simulink model "FaultCheck"  (R2022b)
settings: Solver=FixedStepAuto  StartTime=0.0  StopTime=10  FixedStep=1  RelTol=1e-3
undefined symbols (not defined in the file): C_Flt_IGBTULowerTempConfirmTh_u16, C_Flt_IGBTULowerTempDiagEn_b, C_Flt_IGBTULowerTempErrCode_u16, C_Flt_IGBTULowerTempPowerCoeff, C_Flt_IGBTULowerTempRecoveryTh_u16, C_Flt_IGBTULowerTempRecTh_s32, C_Flt_IGBTULowerTempTrigTh_s32, C_Flt_IGBTUOverTempConfirmTh_u16, C_Flt_IGBTUOverTempDiagEn_b, C_Flt_IGBTUOverTempErrCode_u16, C_Flt_IGBTUOverTempRecoveryTh_u16, C_Flt_IGBTUOverTempRecTh_s32, C_Flt_IGBTUOverTempTrigTh_s32, C_Flt_IGBTVLowerTempConfirmTh_u16, C_Flt_IGBTVLowerTempDiagEn_b, C_Flt_IGBTVLowerTempErrCode_u16, C_Flt_IGBTVLowerTempPowerCoeff, C_Flt_IGBTVLowerTempRecoveryTh_u16, C_Flt_IGBTVLowerTempRecTh_s32, C_Flt_IGBTVLowerTempTrigTh_s32, C_Flt_IGBTVOverTempConfirmTh_u16, C_Flt_IGBTVOverTempDiagEn_b, C_Flt_IGBTVOverTempErrCode_u16, C_Flt_IGBTVOverTempRecoveryTh_u16, C_Flt_IGBTVOverTempRecTh_s32, C_Flt_IGBTVOverTempTrigTh_s32, C_Flt_IGBTWLowerTempConfirmTh_u16, C_Flt_IGBTWLowerTempDiagEn_b, C_Flt_IGBTWLowerTempErrCode_u16, C_Flt_IGBTWLowerTempPowerCoeff, C_Flt_IGBTWLowerTempRecoveryTh_u16, C_Flt_IGBTWLowerTempRecTh_s32, C_Flt_IGBTWLowerTempTrigTh_s32, C_Flt_IGBTWOverTempConfirmTh_u16, C_Flt_IGBTWOverTempDiagEn_b, C_Flt_IGBTWOverTempErrCode_u16, C_Flt_IGBTWOverTempRecoveryTh_u16, C_Flt_IGBTWOverTempRecTh_s32, C_Flt_IGBTWOverTempTrigTh_s32, C_Flt_IuOCConfirmTh_u16, C_Flt_IuOCDiagEn_b, C_Flt_IuOCErrCode_u16, C_Flt_IuOCNegLimit_s32, C_Flt_IuOCPosLimit_s32, C_Flt_IuOCRecoveryTh_u16, C_Flt_IuZeroDriftDiagEn_b, C_Flt_IuZeroDriftErrCode_u16, C_Flt_IvOCConfirmTh_u16, C_Flt_IvOCDiagEn_b, C_Flt_IvOCErrCode_u16, C_Flt_IvOCNegLimit_s32, C_Flt_IvOCPosLimit_s32, C_Flt_IvOCRecoveryTh_u16, C_Flt_IvZeroDriftDiagEn_b, C_Flt_IvZeroDriftErrCode_u16, C_Flt_IwOCConfirmTh_u16, C_Flt_IwOCDiagEn_b, C_Flt_IwOCErrCode_u16, C_Flt_IwOCNegLimit_s32, C_Flt_IwOCPosLimit_s32 ... (+196)
libraries: YS_UserDefined_Library x21, simulink x5
(part 7 of 11)

== system FaultCheck/FaultDiag_HighTask_100us/FltDetn/RecUDetn/RecUDetn/FltLvl ==
  note: SWFD--ComReq-01-09
      | SWFD--ComReq-01-10
      | SWFD--ComReq-01-11
      | SWFD--ComReq-01-12
  ErrDetnFlgOut : Inport
  FltLvl : Inport  Port=2
  If : If  IfExpression=u1==0
  If Action Subsystem : Subsystem  TreatAsAtomicUnit=on
  If Action Subsystem1 : Subsystem  TreatAsAtomicUnit=on
  Merge : Merge
  Flt_RecUFltLvl : Outport
  wires:
  If Action Subsystem1/1(ValOut) -> Merge/2
  FltLvl/1 -> If Action Subsystem1/1(In)
  ErrDetnFlgOut/1 -> If/1
  If/2 -> If Action Subsystem1/Action
  If/1 -> If Action Subsystem/Action
  Merge/1 -> Flt_RecUFltLvl/1  "Flt_RecUFltLvl"
  If Action Subsystem/1(ValOut) -> Merge/1

== system FaultCheck/FaultDiag_HighTask_100us/FltDetn/RecUDetn/RecUDetn/Power Reduction Coefficient ==
  note: SWFD--ComReq-01-06
      | SWFD--ComReq-01-07
      | SWFD--ComReq-01-08
      | SWFD--ComReq-01-09
  FltLvlOut : Inport
  PowRecCoef : Inport  Port=2
  If : If  IfExpression=u1<2  ElseIfExpressions=u1==2
  If Action Subsystem : Subsystem  TreatAsAtomicUnit=on
  If Action Subsystem1 : Subsystem  TreatAsAtomicUnit=on
  If Action Subsystem2 : Subsystem  TreatAsAtomicUnit=on
  Merge : Merge  Inputs=3
  Flt_RecUPowRecCoefOut : Outport
  wires:
  If/1 -> If Action Subsystem/Action
  If Action Subsystem2/1(PowRecCoefOut) -> Merge/3
  If/3 -> If Action Subsystem2/Action
  FltLvlOut/1 -> If/1
  PowRecCoef/1 -> If Action Subsystem1/1(PowRecCoef)
  If Action Subsystem1/1(PowRecCoefOut) -> Merge/2
  If Action Subsystem/1(PowRecCoefOut) -> Merge/1
  Merge/1 -> Flt_RecUPowRecCoefOut/1  "Flt_RecUPowRecCoefOut"
  If/2 -> If Action Subsystem1/Action

== system FaultCheck/FaultDiag_HighTask_100us/FltDetn/RecUDetn/RecUDetn/Subsystem ==
  note: SWFD--ComReq-01-14
  Flt_RecUErrFlg : Inport
  InPutVal : Inport  Port=2
  Constant : Constant  Value=Flt_RecUSubValue
  Switch : Switch  Criteria=u2 > Threshold  SaturateOnIntegerOverflow=off  InputSameDT=off
  Flt_RecUFin : Outport
  wires:
  Constant/1 -> Switch/1
  Switch/1 -> Flt_RecUFin/1
  InPutVal/1 -> Switch/3
  Flt_RecUErrFlg/1 -> Switch/2

== system FaultCheck/FaultDiag_HighTask_100us/FltDetn/ResErrFlgDetn/ResErrDetn/ErrCode ==
  ErrDetnFlgOut : Inport
  ErrCode : Inport  Port=2
  If : If  IfExpression=u1==0
  If Action Subsystem : Subsystem  TreatAsAtomicUnit=on
  If Action Subsystem1 : Subsystem  TreatAsAtomicUnit=on
  wires:
  ErrDetnFlgOut/1 -> If/1
  If/2 -> If Action Subsystem1/Action
  If/1 -> If Action Subsystem/Action
  ErrCode/1 -> If Action Subsystem1/1(ErrCod)

== system FaultCheck/FaultDiag_HighTask_100us/FltDetn/ResErrFlgDetn/ResErrDetn/ErrDetn ==
  InputVal : Inport
  EnabDetn : Inport  Port=2
  ActvnDetn : Inport  Port=3
  AND1 : Logic  AllPortsSameDT=off  OutDataTypeStr=boolean
  Constant10 : Constant  Value=FLT_ON
  Constant9 : Constant  Value=FLT_ON
  If : If  IfExpression=u1 == 0
  If Action Subsystem : Subsystem  TreatAsAtomicUnit=on
  If Action Subsystem1 : Subsystem  TreatAsAtomicUnit=on
  Merge : Merge
  Relational Operator3 : RelationalOperator  Operator===  OutDataTypeStr=boolean  RndMeth=Simplest  InputSameDT=off
  Relational Operator4 : RelationalOperator  Operator===  OutDataTypeStr=boolean  RndMeth=Simplest  InputSameDT=off
  Flt_ResErrErrFlg : Outport
  wires:
  InputVal/1 -> If Action Subsystem1/1(InputVal)
  Merge/1 -> Flt_ResErrErrFlg/1  "Flt_ResErrErrFlg"
  If Action Subsystem/1(Out1) -> Merge/1
  If Action Subsystem1/1(Out1) -> Merge/2
  If/2 -> If Action Subsystem1/Action
  If/1 -> If Action Subsystem/Action
  AND1/1 -> If/1
  Relational Operator4/1 -> AND1/2
  Constant9/1 -> Relational Operator3/2
  Relational Operator3/1 -> AND1/1
  EnabDetn/1 -> Relational Operator4/2
  Constant10/1 -> Relational Operator4/1
  ActvnDetn/1 -> Relational Operator3/1

== system FaultCheck/FaultDiag_HighTask_100us/FltDetn/ResErrFlgDetn/ResErrDetn/FltLvl ==
  ErrDetnFlgOut : Inport
  FltLvl : Inport  Port=2
  If : If  IfExpression=u1==0
  If Action Subsystem : Subsystem  TreatAsAtomicUnit=on
  If Action Subsystem1 : Subsystem  TreatAsAtomicUnit=on
  Merge : Merge
  Flt_ResErrFltLvl : Outport
  wires:
  If Action Subsystem1/1(ValOut) -> Merge/2
  FltLvl/1 -> If Action Subsystem1/1(In)
  ErrDetnFlgOut/1 -> If/1
  If/2 -> If Action Subsystem1/Action
  If/1 -> If Action Subsystem/Action
  Merge/1 -> Flt_ResErrFltLvl/1  "Flt_ResErrFltLvl"
  If Action Subsystem/1(ValOut) -> Merge/1

== system FaultCheck/FaultDiag_HighTask_100us/FltDetn/ResErrFlgDetn/ResErrDetn/Power Reduction Coefficient ==
  FltLvlOut : Inport
  PowRecCoef : Inport  Port=2
  If : If  IfExpression=u1<2  ElseIfExpressions=u1==2
  If Action Subsystem : Subsystem  TreatAsAtomicUnit=on
  If Action Subsystem1 : Subsystem  TreatAsAtomicUnit=on
  If Action Subsystem2 : Subsystem  TreatAsAtomicUnit=on
  Merge : Merge  Inputs=3
  Flt_ResErrPowRecCoefOut : Outport
  wires:
  If/2 -> If Action Subsystem1/Action
  Merge/1 -> Flt_ResErrPowRecCoefOut/1  "Flt_ResErrPowRecCoefOut"
  If Action Subsystem/1(PowRecCoefOut) -> Merge/1
  If Action Subsystem1/1(PowRecCoefOut) -> Merge/2
  PowRecCoef/1 -> If Action Subsystem1/1(PowRecCoef)
  FltLvlOut/1 -> If/1
  If/3 -> If Action Subsystem2/Action
  If Action Subsystem2/1(PowRecCoefOut) -> Merge/3
  If/1 -> If Action Subsystem/Action

== system FaultCheck/FaultDiag_HighTask_100us/FltDetn/ResolveSensorDetn/Flt_ResolveSensorDetn/ErrCode ==
  note: SWFD--ComReq-01-13
  ErrDetnFlgOut : Inport
  ErrCode : Inport  Port=2
  If : If  IfExpression=u1==0
  If Action Subsystem : Subsystem  TreatAsAtomicUnit=on
  If Action Subsystem1 : Subsystem  TreatAsAtomicUnit=on
  wires:
  ErrCode/1 -> If Action Subsystem1/1(ErrCod)
  If/1 -> If Action Subsystem/Action
  If/2 -> If Action Subsystem1/Action
  ErrDetnFlgOut/1 -> If/1

== system FaultCheck/FaultDiag_HighTask_100us/FltDetn/ResolveSensorDetn/Flt_ResolveSensorDetn/ErrDetn ==
  InputVal : Inport
  EnabDetn : Inport  Port=2
  ActvnDetn : Inport  Port=3
  ErrDeb : Inport  Port=4
  AND1 : Logic  AllPortsSameDT=off  OutDataTypeStr=boolean
  Constant10 : Constant  Value=FLT_ON
  Constant9 : Constant  Value=FLT_ON
  If : If  IfExpression=u1 == 0
  If Action Subsystem : Subsystem  TreatAsAtomicUnit=on
  If Action Subsystem1 : Subsystem  TreatAsAtomicUnit=on
  Merge : Merge
  Relational Operator3 : RelationalOperator  Operator===  OutDataTypeStr=boolean  RndMeth=Simplest  InputSameDT=off
  Relational Operator4 : RelationalOperator  Operator===  OutDataTypeStr=boolean  RndMeth=Simplest  InputSameDT=off
  Flt_ResolveSensorErrFlg : Outport
  wires:
  InputVal/1 -> If Action Subsystem1/1(InputVal)
  ActvnDetn/1 -> Relational Operator3/1
  Constant10/1 -> Relational Operator4/1
  EnabDetn/1 -> Relational Operator4/2
  Relational Operator3/1 -> AND1/1
  Constant9/1 -> Relational Operator3/2
  Relational Operator4/1 -> AND1/2
  AND1/1 -> If/1
  If/1 -> If Action Subsystem/Action
  If/2 -> If Action Subsystem1/Action
  If Action Subsystem1/1(Out1) -> Merge/2
  If Action Subsystem/1(Out1) -> Merge/1
  Merge/1 -> Flt_ResolveSensorErrFlg/1
  ErrDeb/1 -> If Action Subsystem1/2(ErrDeb)

== system FaultCheck/FaultDiag_HighTask_100us/FltDetn/ResolveSensorDetn/Flt_ResolveSensorDetn/FltLvl ==
  note: SWFD--ComReq-01-09
      | SWFD--ComReq-01-10
      | SWFD--ComReq-01-11
      | SWFD--ComReq-01-12
  ErrDetnFlgOut : Inport
  FltLvl : Inport  Port=2
  If : If  IfExpression=u1==0
  If Action Subsystem : Subsystem  TreatAsAtomicUnit=on
  If Action Subsystem1 : Subsystem  TreatAsAtomicUnit=on
  Merge : Merge
  Flt_ResolveSensorFltLvl : Outport
  wires:
  If Action Subsystem/1(ValOut) -> Merge/1
  Merge/1 -> Flt_ResolveSensorFltLvl/1  "Flt_ResolveSensorFltLvl"
  If/1 -> If Action Subsystem/Action
  If/2 -> If Action Subsystem1/Action
  ErrDetnFlgOut/1 -> If/1
  FltLvl/1 -> If Action Subsystem1/1(In)
  If Action Subsystem1/1(ValOut) -> Merge/2

== system FaultCheck/FaultDiag_HighTask_100us/FltDetn/ResolveSensorDetn/Flt_ResolveSensorDetn/Power Reduction Coefficient ==
  note: SWFD--ComReq-01-06
      | SWFD--ComReq-01-07
      | SWFD--ComReq-01-08
      | SWFD--ComReq-01-09
  FltLvlOut : Inport
  PowRecCoef : Inport  Port=2
  If : If  IfExpression=u1<2  ElseIfExpressions=u1==2
  If Action Subsystem : Subsystem  TreatAsAtomicUnit=on
  If Action Subsystem1 : Subsystem  TreatAsAtomicUnit=on
  If Action Subsystem2 : Subsystem  TreatAsAtomicUnit=on
  Merge : Merge  Inputs=3
  Flt_ResolveSensorPowRecCoefOut : Outport
  wires:
  If/1 -> If Action Subsystem/Action
  If Action Subsystem2/1(PowRecCoefOut) -> Merge/3
  If/3 -> If Action Subsystem2/Action
  FltLvlOut/1 -> If/1
  PowRecCoef/1 -> If Action Subsystem1/1(PowRecCoef)
  If Action Subsystem1/1(PowRecCoefOut) -> Merge/2
  If Action Subsystem/1(PowRecCoefOut) -> Merge/1
  Merge/1 -> Flt_ResolveSensorPowRecCoefOut/1  "Flt_ResolveSensorPowRecCoefOut"
  If/2 -> If Action Subsystem1/Action

== system FaultCheck/FaultDiag_HighTask_100us/FltDetn/UdcDetn/UdcOverLim1Detn/ErrCode1 ==
  note: SWFD--ComReq-01-13
  ErrDetnFlgOut : Inport
  ErrCode : Inport  Port=2
  If : If  IfExpression=u1==0
  If Action Subsystem : Subsystem  TreatAsAtomicUnit=on
  If Action Subsystem1 : Subsystem  TreatAsAtomicUnit=on
  wires:
  ErrCode/1 -> If Action Subsystem1/1(ErrCod)
  If/1 -> If Action Subsystem/Action
  If/2 -> If Action Subsystem1/Action
  ErrDetnFlgOut/1 -> If/1

== system FaultCheck/FaultDiag_HighTask_100us/FltDetn/UdcDetn/UdcOverLim1Detn/ErrDetn ==
  InputVal : Inport
  EnabDetn : Inport  Port=2
  ActvnDetn : Inport  Port=3
  OverLim1 : Inport  Port=4
  CntrRecLim : Inport  Port=5
  RecLim1 : Inport  Port=6
  CntrFltLim : Inport  Port=7
  AND1 : Logic  AllPortsSameDT=off  OutDataTypeStr=boolean
  Constant10 : Constant  Value=FLT_ON
  Constant9 : Constant  Value=FLT_ON
  If : If  IfExpression=u1 == 0
  If Action Subsystem : Subsystem  TreatAsAtomicUnit=on
  If Action Subsystem1 : Subsystem  TreatAsAtomicUnit=on
  Merge : Merge
  Relational Operator3 : RelationalOperator  Operator===  OutDataTypeStr=boolean  RndMeth=Simplest  InputSameDT=off
  Relational Operator4 : RelationalOperator  Operator===  OutDataTypeStr=boolean  RndMeth=Simplest  InputSameDT=off
  Flt_UdcOverLim1ErrDetnFlg : Outport
  wires:
  ActvnDetn/1 -> Relational Operator3/1
  Constant10/1 -> Relational Operator4/1
  EnabDetn/1 -> Relational Operator4/2
  Relational Operator3/1 -> AND1/1
  Constant9/1 -> Relational Operator3/2
  Relational Operator4/1 -> AND1/2
  AND1/1 -> If/1
  If/1 -> If Action Subsystem/Action
  If/2 -> If Action Subsystem1/Action
  If Action Subsystem/1(Out1) -> Merge/1
  Merge/1 -> Flt_UdcOverLim1ErrDetnFlg/1  "Flt_UdcOverLim1ErrDetnFlg"
  InputVal/1 -> If Action Subsystem1/1(InputVal)
  OverLim1/1 -> If Action Subsystem1/2(OverLim1)
  CntrRecLim/1 -> If Action Subsystem1/5(CntrRecLim)
  If Action Subsystem1/1(FltFlg) -> Merge/2
  RecLim1/1 -> If Action Subsystem1/3(RecLim1)
  CntrFltLim/1 -> If Action Subsystem1/4(CntrFltLim)

== system FaultCheck/FaultDiag_HighTask_100us/FltDetn/UdcDetn/UdcOverLim1Detn/FltLvl ==
  note: SWFD--ComReq-01-09
      | SWFD--ComReq-01-10
      | SWFD--ComReq-01-11
      | SWFD--ComReq-01-12
  ErrDetnFlgOut : Inport
  FltLvl : Inport  Port=2
  If : If  IfExpression=u1==0
  If Action Subsystem : Subsystem  TreatAsAtomicUnit=on
  If Action Subsystem1 : Subsystem  TreatAsAtomicUnit=on
  Merge : Merge
  Flt_UdcOverLim1FltLvlOut : Outport
  wires:
  If Action Subsystem/1(ValOut) -> Merge/1
  Merge/1 -> Flt_UdcOverLim1FltLvlOut/1  "Flt_UdcOverLim1FltLvlOut"
  If/1 -> If Action Subsystem/Action
  If/2 -> If Action Subsystem1/Action
  ErrDetnFlgOut/1 -> If/1
  FltLvl/1 -> If Action Subsystem1/1(In)
  If Action Subsystem1/1(ValOut) -> Merge/2

== system FaultCheck/FaultDiag_HighTask_100us/FltDetn/UdcDetn/UdcOverLim1Detn/Power Reduction Coefficient ==
  note: SWFD--ComReq-01-06
      | SWFD--ComReq-01-07
      | SWFD--ComReq-01-08
      | SWFD--ComReq-01-09
  FltLvlOut : Inport
  PowRecCoef : Inport  Port=2
  If : If  IfExpression=u1<2  ElseIfExpressions=u1==2
  If Action Subsystem : Subsystem  TreatAsAtomicUnit=on
  If Action Subsystem1 : Subsystem  TreatAsAtomicUnit=on
  If Action Subsystem2 : Subsystem  TreatAsAtomicUnit=on
  Merge : Merge  Inputs=3
  Flt_UdcOverLim1RecCoefOut : Outport
  wires:
  If/2 -> If Action Subsystem1/Action
  If/3 -> If Action Subsystem2/Action
  If/1 -> If Action Subsystem/Action
  If Action Subsystem2/1(PowRecCoefOut) -> Merge/3
  FltLvlOut/1 -> If/1
  PowRecCoef/1 -> If Action Subsystem1/1(PowRecCoef)
  If Action Subsystem1/1(PowRecCoefOut) -> Merge/2
  If Action Subsystem/1(PowRecCoefOut) -> Merge/1
  Merge/1 -> Flt_UdcOverLim1RecCoefOut/1  "Flt_UdcOverLim1RecCoefOut"

== system FaultCheck/FaultDiag_HighTask_100us/FltDetn/UdcDetn/UdcOverLim1Detn/Subsystem ==
  note: SWFD--ComReq-01-14
  Flt_UdcOverLim1ErrDetnFlg : Inport
  InPutVal : Inport  Port=2
  Constant : Constant  Value=Flt_UdcOverLim1SubValue
  Switch : Switch  Criteria=u2 > Threshold  SaturateOnIntegerOverflow=off  InputSameDT=off
  Flt_UdcOverLim1Fin : Outport
  wires:
  Constant/1 -> Switch/1
  Switch/1 -> Flt_UdcOverLim1Fin/1
  InPutVal/1 -> Switch/3
  Flt_UdcOverLim1ErrDetnFlg/1 -> Switch/2

== system FaultCheck/FaultDiag_HighTask_100us/FltDetn/UdcDetn/UdcOverLim2Detn/ErrCode1 ==
  note: SWFD--ComReq-01-13
  ErrDetnFlgOut : Inport
  ErrCode : Inport  Port=2
  If : If  IfExpression=u1==0
  If Action Subsystem : Subsystem  TreatAsAtomicUnit=on
  If Action Subsystem1 : Subsystem  TreatAsAtomicUnit=on
  wires:
  ErrCode/1 -> If Action Subsystem1/1(ErrCod)
  If/1 -> If Action Subsystem/Action
  If/2 -> If Action Subsystem1/Action
  ErrDetnFlgOut/1 -> If/1

== system FaultCheck/FaultDiag_HighTask_100us/FltDetn/UdcDetn/UdcOverLim2Detn/ErrDetn ==
  InputVal : Inport
  EnabDetn : Inport  Port=2
  ActvnDetn : Inport  Port=3
  CntrFltLim : Inport  Port=4
  OverLim2 : Inport  Port=5
  AND1 : Logic  AllPortsSameDT=off  OutDataTypeStr=boolean
  Constant10 : Constant  Value=FLT_ON
  Constant9 : Constant  Value=FLT_ON
  If : If  IfExpression=u1 == 0
  If Action Subsystem : Subsystem  TreatAsAtomicUnit=on
  If Action Subsystem1 : Subsystem  TreatAsAtomicUnit=on
  Merge : Merge
  Relational Operator1 : RelationalOperator  OutDataTypeStr=boolean  RndMeth=Simplest  InputSameDT=off
  Relational Operator3 : RelationalOperator  Operator===  OutDataTypeStr=boolean  RndMeth=Simplest  InputSameDT=off
  Relational Operator4 : RelationalOperator  Operator===  OutDataTypeStr=boolean  RndMeth=Simplest  InputSameDT=off
  Flt_UdcOverLim2ErrDetnFlg : Outport
  wires:
  Relational Operator1/1 -> If Action Subsystem1/1(InputVal)
  InputVal/1 -> Relational Operator1/1
  OverLim2/1 -> Relational Operator1/2
  CntrFltLim/1 -> If Action Subsystem1/2(ErrDeb)
  If Action Subsystem1/1(Out1) -> Merge/2
  Merge/1 -> Flt_UdcOverLim2ErrDetnFlg/1  "Flt_UdcOverLim2ErrDetnFlg"
  If Action Subsystem/1(Out1) -> Merge/1
  If/2 -> If Action Subsystem1/Action
  If/1 -> If Action Subsystem/Action
  AND1/1 -> If/1
  Relational Operator4/1 -> AND1/2
  Constant9/1 -> Relational Operator3/2
  Relational Operator3/1 -> AND1/1
  EnabDetn/1 -> Relational Operator4/2
  Constant10/1 -> Relational Operator4/1
  ActvnDetn/1 -> Relational Operator3/1

== system FaultCheck/FaultDiag_HighTask_100us/FltDetn/UdcDetn/UdcOverLim2Detn/FltLvl ==
  note: SWFD--ComReq-01-09
      | SWFD--ComReq-01-10
      | SWFD--ComReq-01-11
      | SWFD--ComReq-01-12
  ErrDetnFlgOut : Inport
  FltLvl : Inport  Port=2
  If : If  IfExpression=u1==0
  If Action Subsystem : Subsystem  TreatAsAtomicUnit=on
  If Action Subsystem1 : Subsystem  TreatAsAtomicUnit=on
  Merge : Merge
  Flt_UdcOverLim2FltLvlOut : Outport
  wires:
  If Action Subsystem1/1(ValOut) -> Merge/2
  FltLvl/1 -> If Action Subsystem1/1(In)
  ErrDetnFlgOut/1 -> If/1
  If/2 -> If Action Subsystem1/Action
  If/1 -> If Action Subsystem/Action
  Merge/1 -> Flt_UdcOverLim2FltLvlOut/1  "Flt_UdcOverLim2FltLvlOut"
  If Action Subsystem/1(ValOut) -> Merge/1

== system FaultCheck/FaultDiag_HighTask_100us/FltDetn/UdcDetn/UdcOverLim2Detn/Power Reduction Coefficient ==
  note: SWFD--ComReq-01-06
      | SWFD--ComReq-01-07
      | SWFD--ComReq-01-08
      | SWFD--ComReq-01-09
  FltLvlOut : Inport
  PowRecCoef : Inport  Port=2
  If : If  IfExpression=u1<2  ElseIfExpressions=u1==2
  If Action Subsystem : Subsystem  TreatAsAtomicUnit=on
  If Action Subsystem1 : Subsystem  TreatAsAtomicUnit=on
  If Action Subsystem2 : Subsystem  TreatAsAtomicUnit=on
  Merge : Merge  Inputs=3
  Flt_UdcOverLim2RecCoefOut : Outport
  wires:
  If/1 -> If Action Subsystem/Action
  If Action Subsystem2/1(PowRecCoefOut) -> Merge/3
  If/3 -> If Action Subsystem2/Action
  FltLvlOut/1 -> If/1
  PowRecCoef/1 -> If Action Subsystem1/1(PowRecCoef)
  If Action Subsystem1/1(PowRecCoefOut) -> Merge/2
  If Action Subsystem/1(PowRecCoefOut) -> Merge/1
  Merge/1 -> Flt_UdcOverLim2RecCoefOut/1  "Flt_UdcOverLim2RecCoefOut"
  If/2 -> If Action Subsystem1/Action

== system FaultCheck/FaultDiag_HighTask_100us/FltDetn/UdcDetn/UdcOverLim2Detn/Subsystem ==
  note: SWFD--ComReq-01-14
  Flt_UdcOverLim2ErrDetnFlg : Inport
  InPutVal : Inport  Port=2
  Constant : Constant  Value=Flt_UdcOverLim2SubValue
  Switch : Switch  Criteria=u2 > Threshold  SaturateOnIntegerOverflow=off  InputSameDT=off
  Flt_UdcOverLim2Fin : Outport
  wires:
  Constant/1 -> Switch/1
  Switch/1 -> Flt_UdcOverLim2Fin/1
  InPutVal/1 -> Switch/3
  Flt_UdcOverLim2ErrDetnFlg/1 -> Switch/2

== system FaultCheck/FaultDiag_HighTask_100us/FltDetn/UdcDetn/UdcUnderLim1Detn/ErrCode1 ==
  note: SWFD--ComReq-01-13
  ErrDetnFlgOut : Inport
  ErrCode : Inport  Port=2
  If : If  IfExpression=u1==0
  If Action Subsystem : Subsystem  TreatAsAtomicUnit=on
  If Action Subsystem1 : Subsystem  TreatAsAtomicUnit=on
  wires:
  ErrCode/1 -> If Action Subsystem1/1(ErrCod)
  If/1 -> If Action Subsystem/Action
  If/2 -> If Action Subsystem1/Action
  ErrDetnFlgOut/1 -> If/1

== system FaultCheck/FaultDiag_HighTask_100us/FltDetn/UdcDetn/UdcUnderLim1Detn/ErrDetn ==
  InputVal : Inport
  EnabDetn : Inport  Port=2
  ActvnDetn : Inport  Port=3
  LoLim1 : Inport  Port=4
  CntrRecLim : Inport  Port=5
  RecLim1 : Inport  Port=6
  CntrFltLim : Inport  Port=7
  AND1 : Logic  AllPortsSameDT=off  OutDataTypeStr=boolean
  Constant10 : Constant  Value=FLT_ON
  Constant9 : Constant  Value=FLT_ON
  If : If  IfExpression=u1 == 0
  If Action Subsystem : Subsystem  TreatAsAtomicUnit=on
  If Action Subsystem1 : Subsystem  TreatAsAtomicUnit=on
  Merge : Merge
  Relational Operator3 : RelationalOperator  Operator===  OutDataTypeStr=boolean  RndMeth=Simplest  InputSameDT=off
  Relational Operator4 : RelationalOperator  Operator===  OutDataTypeStr=boolean  RndMeth=Simplest  InputSameDT=off
  Flt_UdcUnderLim1ErrDetnFlg : Outport
  wires:
  CntrFltLim/1 -> If Action Subsystem1/4(CntrFltLim)
  RecLim1/1 -> If Action Subsystem1/3(RecLim1)
  If Action Subsystem1/1(FltFlg) -> Merge/2
  CntrRecLim/1 -> If Action Subsystem1/5(CntrRecLim)
  LoLim1/1 -> If Action Subsystem1/2(LoLim1)
  InputVal/1 -> If Action Subsystem1/1(InputVal)
  Merge/1 -> Flt_UdcUnderLim1ErrDetnFlg/1  "Flt_UdcUnderLim1ErrDetnFlg"
  If Action Subsystem/1(Out1) -> Merge/1
  If/2 -> If Action Subsystem1/Action
  If/1 -> If Action Subsystem/Action
  AND1/1 -> If/1
  Relational Operator4/1 -> AND1/2
  Constant9/1 -> Relational Operator3/2
  Relational Operator3/1 -> AND1/1
  EnabDetn/1 -> Relational Operator4/2
  Constant10/1 -> Relational Operator4/1
  ActvnDetn/1 -> Relational Operator3/1

== system FaultCheck/FaultDiag_HighTask_100us/FltDetn/UdcDetn/UdcUnderLim1Detn/FltLvl ==
  note: SWFD--ComReq-01-09
      | SWFD--ComReq-01-10
      | SWFD--ComReq-01-11
      | SWFD--ComReq-01-12
  ErrDetnFlgOut : Inport
  FltLvl : Inport  Port=2
  If : If  IfExpression=u1==0
  If Action Subsystem : Subsystem  TreatAsAtomicUnit=on
  If Action Subsystem1 : Subsystem  TreatAsAtomicUnit=on
  Merge : Merge
  Flt_UdcUnderLim1FltLvlOut : Outport
  wires:
  If Action Subsystem1/1(ValOut) -> Merge/2
  FltLvl/1 -> If Action Subsystem1/1(In)
  ErrDetnFlgOut/1 -> If/1
  If/2 -> If Action Subsystem1/Action
  If/1 -> If Action Subsystem/Action
  Merge/1 -> Flt_UdcUnderLim1FltLvlOut/1  "Flt_UdcUnderLim1FltLvlOut"
  If Action Subsystem/1(ValOut) -> Merge/1

== system FaultCheck/FaultDiag_HighTask_100us/FltDetn/UdcDetn/UdcUnderLim1Detn/Power Reduction Coefficient ==
  note: SWFD--ComReq-01-06
      | SWFD--ComReq-01-07
      | SWFD--ComReq-01-08
      | SWFD--ComReq-01-09
  FltLvlOut : Inport
  PowRecCoef : Inport  Port=2
  If : If  IfExpression=u1<2  ElseIfExpressions=u1==2
  If Action Subsystem : Subsystem  TreatAsAtomicUnit=on
  If Action Subsystem1 : Subsystem  TreatAsAtomicUnit=on
  If Action Subsystem2 : Subsystem  TreatAsAtomicUnit=on
  Merge : Merge  Inputs=3
  Flt_UdcUnderLim1RecCoefOut : Outport
  wires:
  If/2 -> If Action Subsystem1/Action
  If/3 -> If Action Subsystem2/Action
  If/1 -> If Action Subsystem/Action
  If Action Subsystem2/1(PowRecCoefOut) -> Merge/3
  FltLvlOut/1 -> If/1
  PowRecCoef/1 -> If Action Subsystem1/1(PowRecCoef)
  If Action Subsystem1/1(PowRecCoefOut) -> Merge/2
  If Action Subsystem/1(PowRecCoefOut) -> Merge/1
  Merge/1 -> Flt_UdcUnderLim1RecCoefOut/1  "Flt_UdcUnderLim1RecCoefOut"

== system FaultCheck/FaultDiag_HighTask_100us/FltDetn/UdcDetn/UdcUnderLim1Detn/Subsystem ==
  note: SWFD--ComReq-01-14
  Flt_UdcUnderLim1ErrDetnFlg : Inport
  InPutVal : Inport  Port=2
  Constant : Constant  Value=Flt_UdcUnderLim1SubValue
  Switch : Switch  Criteria=u2 > Threshold  SaturateOnIntegerOverflow=off  InputSameDT=off
  Flt_UdcUnderLim1Fin : Outport
  wires:
  Constant/1 -> Switch/1
  Switch/1 -> Flt_UdcUnderLim1Fin/1
  InPutVal/1 -> Switch/3
  Flt_UdcUnderLim1ErrDetnFlg/1 -> Switch/2

== system FaultCheck/FaultDiag_HighTask_100us/FltDetn/UdcDetn/UdcUnderLim2Detn2/ErrCode1 ==
  note: SWFD--ComReq-01-13
  ErrDetnFlgOut : Inport
  ErrCode : Inport  Port=2
  If : If  IfExpression=u1==0
  If Action Subsystem : Subsystem  TreatAsAtomicUnit=on
  If Action Subsystem1 : Subsystem  TreatAsAtomicUnit=on
  wires:
  ErrCode/1 -> If Action Subsystem1/1(ErrCod)
  If/1 -> If Action Subsystem/Action
  If/2 -> If Action Subsystem1/Action
  ErrDetnFlgOut/1 -> If/1

== system FaultCheck/FaultDiag_HighTask_100us/FltDetn/UdcDetn/UdcUnderLim2Detn2/ErrDetn ==
  InputVal : Inport
  EnabDetn : Inport  Port=2
  ActvnDetn : Inport  Port=3
  LoLim2 : Inport  Port=4
  CntrRecLim : Inport  Port=5
  RecLim2 : Inport  Port=6
  CntrFltLim : Inport  Port=7
  AND1 : Logic  AllPortsSameDT=off  OutDataTypeStr=boolean
  Constant10 : Constant  Value=FLT_ON
  Constant9 : Constant  Value=FLT_ON
  If : If  IfExpression=u1 == 0
  If Action Subsystem : Subsystem  TreatAsAtomicUnit=on
  If Action Subsystem1 : Subsystem  TreatAsAtomicUnit=on
  Merge : Merge
  Relational Operator3 : RelationalOperator  Operator===  OutDataTypeStr=boolean  RndMeth=Simplest  InputSameDT=off
  Relational Operator4 : RelationalOperator  Operator===  OutDataTypeStr=boolean  RndMeth=Simplest  InputSameDT=off
  Flt_UdcUnderLim2ErrDetnFlg : Outport
  wires:
  ActvnDetn/1 -> Relational Operator3/1
  Constant10/1 -> Relational Operator4/1
  EnabDetn/1 -> Relational Operator4/2
  Relational Operator3/1 -> AND1/1
  Constant9/1 -> Relational Operator3/2
  Relational Operator4/1 -> AND1/2
  AND1/1 -> If/1
  If/1 -> If Action Subsystem/Action
  If/2 -> If Action Subsystem1/Action
  If Action Subsystem/1(Out1) -> Merge/1
  Merge/1 -> Flt_UdcUnderLim2ErrDetnFlg/1  "Flt_UdcUnderLim2ErrDetnFlg"
  InputVal/1 -> If Action Subsystem1/1(InputVal)
  LoLim2/1 -> If Action Subsystem1/2(LoLim2)
  CntrRecLim/1 -> If Action Subsystem1/5(CntrRecLim)
  If Action Subsystem1/1(FltFlg) -> Merge/2
  RecLim2/1 -> If Action Subsystem1/3(RecLim2)
  CntrFltLim/1 -> If Action Subsystem1/4(CntrFltLim)

== system FaultCheck/FaultDiag_HighTask_100us/FltDetn/UdcDetn/UdcUnderLim2Detn2/FltLvl ==
  note: SWFD--ComReq-01-09
      | SWFD--ComReq-01-10
      | SWFD--ComReq-01-11
      | SWFD--ComReq-01-12
  ErrDetnFlgOut : Inport
  FltLvl : Inport  Port=2
  If : If  IfExpression=u1==0
  If Action Subsystem : Subsystem  TreatAsAtomicUnit=on
  If Action Subsystem1 : Subsystem  TreatAsAtomicUnit=on
  Merge : Merge
  Flt_UdcUnderLim2FltLvlOut : Outport
  wires:
  If Action Subsystem/1(ValOut) -> Merge/1
  Merge/1 -> Flt_UdcUnderLim2FltLvlOut/1  "Flt_UdcUnderLim2FltLvlOut"
  If/1 -> If Action Subsystem/Action
  If/2 -> If Action Subsystem1/Action
  ErrDetnFlgOut/1 -> If/1
  FltLvl/1 -> If Action Subsystem1/1(In)
  If Action Subsystem1/1(ValOut) -> Merge/2

== system FaultCheck/FaultDiag_HighTask_100us/FltDetn/UdcDetn/UdcUnderLim2Detn2/Power Reduction Coefficient ==
  note: SWFD--ComReq-01-06
      | SWFD--ComReq-01-07
      | SWFD--ComReq-01-08
      | SWFD--ComReq-01-09
  FltLvlOut : Inport
  PowRecCoef : Inport  Port=2
  If : If  IfExpression=u1<2  ElseIfExpressions=u1==2
  If Action Subsystem : Subsystem  TreatAsAtomicUnit=on
  If Action Subsystem1 : Subsystem  TreatAsAtomicUnit=on
  If Action Subsystem2 : Subsystem  TreatAsAtomicUnit=on
  Merge : Merge  Inputs=3
  Flt_UdcUnderLim2RecCoefOut : Outport
  wires:
  If/2 -> If Action Subsystem1/Action
  If/3 -> If Action Subsystem2/Action
  If/1 -> If Action Subsystem/Action
  If Action Subsystem2/1(PowRecCoefOut) -> Merge/3
  FltLvlOut/1 -> If/1
  PowRecCoef/1 -> If Action Subsystem1/1(PowRecCoef)
  If Action Subsystem1/1(PowRecCoefOut) -> Merge/2
  If Action Subsystem/1(PowRecCoefOut) -> Merge/1
  Merge/1 -> Flt_UdcUnderLim2RecCoefOut/1  "Flt_UdcUnderLim2RecCoefOut"

== system FaultCheck/FaultDiag_HighTask_100us/FltDetn/UdcDetn/UdcUnderLim2Detn2/Subsystem ==
  note: SWFD--ComReq-01-14
  Flt_UdcUnderLim2ErrDetnFlg : Inport
  InPutVal : Inport  Port=2
  Constant : Constant  Value=Flt_UdcUnderLim2SubValue
  Switch : Switch  Criteria=u2 > Threshold  SaturateOnIntegerOverflow=off  InputSameDT=off
  Flt_UdcUnderLim2Fin : Outport
  wires:
  Constant/1 -> Switch/1
  Switch/1 -> Flt_UdcUnderLim2Fin/1
  InPutVal/1 -> Switch/3
  Flt_UdcUnderLim2ErrDetnFlg/1 -> Switch/2

== system FaultCheck/FaultDiag_HighTask_100us/FltDetn/UdcZeroDrfDetn/UdcZeroDrfDetn/ErrCode1 ==
  ErrDetnFlgOut : Inport
  ErrCode : Inport  Port=2
  If : If  IfExpression=u1==0
  If Action Subsystem : Subsystem  TreatAsAtomicUnit=on
  If Action Subsystem1 : Subsystem  TreatAsAtomicUnit=on
  wires:
  ErrDetnFlgOut/1 -> If/1
  If/2 -> If Action Subsystem1/Action
  If/1 -> If Action Subsystem/Action
  ErrCode/1 -> If Action Subsystem1/1(ErrCod)

== system FaultCheck/FaultDiag_HighTask_100us/FltDetn/UdcZeroDrfDetn/UdcZeroDrfDetn/ErrDetn ==
  InputVal : Inport
  EnabDetn : Inport  Port=2
  ActvnDetn : Inport  Port=3
  AND1 : Logic  AllPortsSameDT=off  OutDataTypeStr=boolean
  Constant10 : Constant  Value=FLT_ON
  Constant9 : Constant  Value=FLT_ON
  If : If  IfExpression=u1 == 0
  If Action Subsystem : Subsystem  TreatAsAtomicUnit=on
  If Action Subsystem1 : Subsystem  TreatAsAtomicUnit=on
  Merge : Merge
  Relational Operator3 : RelationalOperator  Operator===  OutDataTypeStr=boolean  RndMeth=Simplest  InputSameDT=off
  Relational Operator4 : RelationalOperator  Operator===  OutDataTypeStr=boolean  RndMeth=Simplest  InputSameDT=off
  Flt_UdcZeroDrfErrFlg : Outport
  wires:
  ActvnDetn/1 -> Relational Operator3/1
  Constant10/1 -> Relational Operator4/1
  EnabDetn/1 -> Relational Operator4/2
  Relational Operator3/1 -> AND1/1
  Constant9/1 -> Relational Operator3/2
  Relational Operator4/1 -> AND1/2
  AND1/1 -> If/1
  If/1 -> If Action Subsystem/Action
  If/2 -> If Action Subsystem1/Action
  If Action Subsystem1/1(Out1) -> Merge/2
  If Action Subsystem/1(Out1) -> Merge/1
  Merge/1 -> Flt_UdcZeroDrfErrFlg/1  "Flt_UdcZeroDrfErrFlg"
  InputVal/1 -> If Action Subsystem1/1(InputVal)

== system FaultCheck/FaultDiag_HighTask_100us/FltDetn/UdcZeroDrfDetn/UdcZeroDrfDetn/FltLvl ==
  ErrDetnFlgOut : Inport
  FltLvl : Inport  Port=2
  If : If  IfExpression=u1==0
  If Action Subsystem : Subsystem  TreatAsAtomicUnit=on
  If Action Subsystem1 : Subsystem  TreatAsAtomicUnit=on
  Merge : Merge
  Flt_UdcZeroDrfFltLvl : Outport
  wires:
  If Action Subsystem/1(ValOut) -> Merge/1
  Merge/1 -> Flt_UdcZeroDrfFltLvl/1  "Flt_UdcZeroDrfFltLv"
  If/1 -> If Action Subsystem/Action
  If/2 -> If Action Subsystem1/Action
  ErrDetnFlgOut/1 -> If/1
  FltLvl/1 -> If Action Subsystem1/1(In)
  If Action Subsystem1/1(ValOut) -> Merge/2

== system FaultCheck/FaultDiag_HighTask_100us/FltDetn/UdcZeroDrfDetn/UdcZeroDrfDetn/Power Reduction Coefficient ==
  FltLvlOut : Inport
  PowRecCoef : Inport  Port=2
  If : If  IfExpression=u1<2  ElseIfExpressions=u1==2
  If Action Subsystem : Subsystem  TreatAsAtomicUnit=on
  If Action Subsystem1 : Subsystem  TreatAsAtomicUnit=on
  If Action Subsystem2 : Subsystem  TreatAsAtomicUnit=on
  Merge : Merge  Inputs=3
  Flt_UdcZeroDrfPowRecCoefOut : Outport
  wires:
  If/2 -> If Action Subsystem1/Action
  Merge/1 -> Flt_UdcZeroDrfPowRecCoefOut/1  "Flt_UdcZeroDrfPowRecCoefOut"
  If Action Subsystem/1(PowRecCoefOut) -> Merge/1
  If Action Subsystem1/1(PowRecCoefOut) -> Merge/2
  PowRecCoef/1 -> If Action Subsystem1/1(PowRecCoef)
  FltLvlOut/1 -> If/1
  If/3 -> If Action Subsystem2/Action
  If Action Subsystem2/1(PowRecCoefOut) -> Merge/3
  If/1 -> If Action Subsystem/Action

== system FaultCheck/FaultDiag_HighTask_100us/FltDetn/VoltagSensorDetn/Flt_VoltagSensorDetn/ErrCode ==
  note: SWFD--ComReq-01-13
  ErrDetnFlgOut : Inport
  ErrCode : Inport  Port=2
  If : If  IfExpression=u1==0
  If Action Subsystem : Subsystem  TreatAsAtomicUnit=on
  If Action Subsystem1 : Subsystem  TreatAsAtomicUnit=on
  wires:
  ErrCode/1 -> If Action Subsystem1/1(ErrCod)
  If/1 -> If Action Subsystem/Action
  If/2 -> If Action Subsystem1/Action
  ErrDetnFlgOut/1 -> If/1

== system FaultCheck/FaultDiag_HighTask_100us/FltDetn/VoltagSensorDetn/Flt_VoltagSensorDetn/ErrDetn ==
  InputVal : Inport
  EnabDetn : Inport  Port=2
  ActvnDetn : Inport  Port=3
  ErrDeb : Inport  Port=4
  AND1 : Logic  AllPortsSameDT=off  OutDataTypeStr=boolean
  Constant10 : Constant  Value=FLT_ON
  Constant9 : Constant  Value=FLT_ON
  If : If  IfExpression=u1 == 0
  If Action Subsystem : Subsystem  TreatAsAtomicUnit=on
  If Action Subsystem1 : Subsystem  TreatAsAtomicUnit=on
  Merge : Merge
  Relational Operator3 : RelationalOperator  Operator===  OutDataTypeStr=boolean  RndMeth=Simplest  InputSameDT=off
  Relational Operator4 : RelationalOperator  Operator===  OutDataTypeStr=boolean  RndMeth=Simplest  InputSameDT=off
  FFlt_VoltagSensorErrFlg : Outport
  wires:
  InputVal/1 -> If Action Subsystem1/1(InputVal)
  ActvnDetn/1 -> Relational Operator3/1
  Constant10/1 -> Relational Operator4/1
  EnabDetn/1 -> Relational Operator4/2
  Relational Operator3/1 -> AND1/1
  Constant9/1 -> Relational Operator3/2
  Relational Operator4/1 -> AND1/2
  AND1/1 -> If/1
  If/1 -> If Action Subsystem/Action
  If/2 -> If Action Subsystem1/Action
  If Action Subsystem1/1(Out1) -> Merge/2
  If Action Subsystem/1(Out1) -> Merge/1
  Merge/1 -> FFlt_VoltagSensorErrFlg/1
  ErrDeb/1 -> If Action Subsystem1/2(ErrDeb)

== system FaultCheck/FaultDiag_HighTask_100us/FltDetn/VoltagSensorDetn/Flt_VoltagSensorDetn/FltLvl ==
  note: SWFD--ComReq-01-09
      | SWFD--ComReq-01-10
      | SWFD--ComReq-01-11
      | SWFD--ComReq-01-12
  ErrDetnFlgOut : Inport
  FltLvl : Inport  Port=2
  If : If  IfExpression=u1==0
  If Action Subsystem : Subsystem  TreatAsAtomicUnit=on
  If Action Subsystem1 : Subsystem  TreatAsAtomicUnit=on
  Merge : Merge
  Flt_VoltagSensorFltLvl : Outport
  wires:
  If Action Subsystem/1(ValOut) -> Merge/1
  Merge/1 -> Flt_VoltagSensorFltLvl/1  "Flt_VoltagSensorFltLvl"
  If/1 -> If Action Subsystem/Action
  If/2 -> If Action Subsystem1/Action
  ErrDetnFlgOut/1 -> If/1
  FltLvl/1 -> If Action Subsystem1/1(In)
  If Action Subsystem1/1(ValOut) -> Merge/2

== system FaultCheck/FaultDiag_HighTask_100us/FltDetn/VoltagSensorDetn/Flt_VoltagSensorDetn/Power Reduction Coefficient ==
  note: SWFD--ComReq-01-06
      | SWFD--ComReq-01-07
      | SWFD--ComReq-01-08
      | SWFD--ComReq-01-09
  FltLvlOut : Inport
  PowRecCoef : Inport  Port=2
  If : If  IfExpression=u1<2  ElseIfExpressions=u1==2
  If Action Subsystem : Subsystem  TreatAsAtomicUnit=on
  If Action Subsystem1 : Subsystem  TreatAsAtomicUnit=on
  If Action Subsystem2 : Subsystem  TreatAsAtomicUnit=on
  Merge : Merge  Inputs=3
  Flt_VoltagSensorPowRecCoefOut : Outport
  wires:
  If/1 -> If Action Subsystem/Action
  If Action Subsystem2/1(PowRecCoefOut) -> Merge/3
  If/3 -> If Action Subsystem2/Action
  FltLvlOut/1 -> If/1
  PowRecCoef/1 -> If Action Subsystem1/1(PowRecCoef)
  If Action Subsystem1/1(PowRecCoefOut) -> Merge/2
  If Action Subsystem/1(PowRecCoefOut) -> Merge/1
  Merge/1 -> Flt_VoltagSensorPowRecCoefOut/1  "Flt_VoltagSensorPowRecCoefOut"
  If/2 -> If Action Subsystem1/Action

== system FaultCheck/FaultDiag_HighTask_100us/FltDetn/VoltagSensorDetn/Flt_VoltagSensorDetn/Subsystem ==
  note: SWFD--ComReq-01-14
  Flt_VoltagSensorErrDetnFlg : Inport
  IPT_UdcRaw_mV : Inport  Port=2
  Constant : Constant  Value=Flt_VoltagSensorSubValue
  Switch : Switch  Criteria=u2 > Threshold  SaturateOnIntegerOverflow=off  InputSameDT=off
  Flt_VoltagSensorFin : Outport
  wires:
  Flt_VoltagSensorErrDetnFlg/1 -> Switch/2
  Constant/1 -> Switch/1
  Switch/1 -> Flt_VoltagSensorFin/1
  IPT_UdcRaw_mV/1 -> Switch/3

== system FaultCheck/FaultDiagnose/CurrZeroDriftFltDiag/IuZeroDriftDiag/Diagnose/Disable ==
  Action Port : ActionPort  ActionPortLabel=if(u1 == 0)
  Constant : Constant  Value=C_Flt_NoErr_b
  FlgOut : Outport
  wires:
  Constant/1 -> FlgOut/1

== system FaultCheck/FaultDiagnose/CurrZeroDriftFltDiag/IuZeroDriftDiag/Diagnose/Normal ==
  IuZeroDriftFltFlg : Inport
  Action Port : ActionPort  ActionPortLabel=else
  Chart : Stateflow chart  TreatAsAtomicUnit=on
  FlgOut : Outport
  wires:
  IuZeroDriftFltFlg/1 -> Chart/1(FltFlg)
  Chart/1(FlgOut) -> FlgOut/1

== system FaultCheck/FaultDiagnose/CurrZeroDriftFltDiag/IuZeroDriftDiag/Diagnose/Subsystem ==
  IuZeroDftEn : Inport
  SysSelfCheckDownFlg : Inport  Port=2
  Constant : Constant  Value=true
  Logical Operator : Logic  AllPortsSameDT=off  OutDataTypeStr=boolean
  Logical Operator1 : Logic  AllPortsSameDT=off  OutDataTypeStr=boolean
  Logical Operator2 : Logic  AllPortsSameDT=off  OutDataTypeStr=boolean
  IuZeroDriftDiagEn : Outport
  wires:
  SysSelfCheckDownFlg/1 -> Logical Operator2/2
  IuZeroDftEn/1 -> Logical Operator1/2
  Logical Operator1/1 -> Logical Operator/1
  Logical Operator2/1 -> Logical Operator/2
  Constant/1 -> Logical Operator1/1, Logical Operator2/1
  Logical Operator/1 -> IuZeroDriftDiagEn/1  "M_Flt_IuZeroDriftDiagEn_b"

== system FaultCheck/FaultDiagnose/CurrZeroDriftFltDiag/IuZeroDriftDiag/FaultLevelDeter/Normal ==
  Action Port : ActionPort  ActionPortLabel=if(u1 == 0)
  Constant : Constant  Value=C_Flt_LevelZero_u8
  IuZeroDriftFltLevel : Outport
  wires:
  Constant/1 -> IuZeroDriftFltLevel/1

== system FaultCheck/FaultDiagnose/CurrZeroDriftFltDiag/IuZeroDriftDiag/FaultLevelDeter/ZeroDriftFlt ==
  FaultLevel : Inport
  Action Port : ActionPort  ActionPortLabel=else
  IuZeroDriftFltLevel : Outport
  wires:
  FaultLevel/1 -> IuZeroDriftFltLevel/1

== system FaultCheck/FaultDiagnose/CurrZeroDriftFltDiag/IuZeroDriftDiag/PowerReductionCoeffDeter/If Action Subsystem ==
  Action Port : ActionPort  ActionPortLabel=if(u1 < 2)
  Constant : Constant  Value=C_Flt_PowerCoeffOne_s32
  Coeff : Outport
  wires:
  Constant/1 -> Coeff/1

== system FaultCheck/FaultDiagnose/CurrZeroDriftFltDiag/IuZeroDriftDiag/PowerReductionCoeffDeter/If Action Subsystem1 ==
  PowerCoeff : Inport
  Action Port : ActionPort  ActionPortLabel=elseif(u1 == 2)
  Coeff : Outport
  wires:
  PowerCoeff/1 -> Coeff/1

== system FaultCheck/FaultDiagnose/CurrZeroDriftFltDiag/IuZeroDriftDiag/PowerReductionCoeffDeter/If Action Subsystem2 ==
  Action Port : ActionPort  ActionPortLabel=else
  Constant : Constant  Value=C_Flt_PowerCoeffZero_s32
  Coeff : Outport
  wires:
  Constant/1 -> Coeff/1

== system FaultCheck/FaultDiagnose/CurrZeroDriftFltDiag/IvZeroDriftDiag/Diagnose/Disable ==
  Action Port : ActionPort  ActionPortLabel=if(u1 == 0)
  Constant : Constant  Value=C_Flt_NoErr_b
  FlgOut : Outport
  wires:
  Constant/1 -> FlgOut/1

== system FaultCheck/FaultDiagnose/CurrZeroDriftFltDiag/IvZeroDriftDiag/Diagnose/Normal ==
  IvZeroDriftFltFlg : Inport
  Action Port : ActionPort  ActionPortLabel=else
  FlgOut : Outport
  wires:
  IvZeroDriftFltFlg/1 -> FlgOut/1

== system FaultCheck/FaultDiagnose/CurrZeroDriftFltDiag/IvZeroDriftDiag/Diagnose/Subsystem ==
  IvZeroDftEn : Inport
  SysSelfCheckDownFlg : Inport  Port=2
  Constant : Constant  Value=true
  Logical Operator : Logic  AllPortsSameDT=off  OutDataTypeStr=boolean
  Logical Operator1 : Logic  AllPortsSameDT=off  OutDataTypeStr=boolean
  Logical Operator2 : Logic  AllPortsSameDT=off  OutDataTypeStr=boolean
  IvZeroDriftDiagEn : Outport
  wires:
  SysSelfCheckDownFlg/1 -> Logical Operator2/2
  IvZeroDftEn/1 -> Logical Operator1/2
  Logical Operator1/1 -> Logical Operator/1
  Logical Operator2/1 -> Logical Operator/2
  Constant/1 -> Logical Operator1/1, Logical Operator2/1
  Logical Operator/1 -> IvZeroDriftDiagEn/1  "M_Flt_IvZeroDriftDiagEn_b"

== system FaultCheck/FaultDiagnose/CurrZeroDriftFltDiag/IvZeroDriftDiag/FaultLevelDeter/Normal ==
  Action Port : ActionPort  ActionPortLabel=if(u1 == 0)
  Constant : Constant  Value=C_Flt_LevelZero_u8
  IvZeroDriftFltLevel : Outport
  wires:
  Constant/1 -> IvZeroDriftFltLevel/1

== system FaultCheck/FaultDiagnose/CurrZeroDriftFltDiag/IvZeroDriftDiag/FaultLevelDeter/ZeroDriftFlt ==
  FaultLevel : Inport
  Action Port : ActionPort  ActionPortLabel=else
  IvZeroDriftFltLevel : Outport
  wires:
  FaultLevel/1 -> IvZeroDriftFltLevel/1

== system FaultCheck/FaultDiagnose/CurrZeroDriftFltDiag/IvZeroDriftDiag/PowerReductionCoeffDeter/If Action Subsystem ==
  Action Port : ActionPort  ActionPortLabel=if(u1 < 2)
  Constant : Constant  Value=C_Flt_PowerCoeffOne_s32
  Coeff : Outport
  wires:
  Constant/1 -> Coeff/1

== system FaultCheck/FaultDiagnose/CurrZeroDriftFltDiag/IvZeroDriftDiag/PowerReductionCoeffDeter/If Action Subsystem1 ==
  PowerCoeff : Inport
  Action Port : ActionPort  ActionPortLabel=elseif(u1 == 2)
  Coeff : Outport
  wires:
  PowerCoeff/1 -> Coeff/1

== system FaultCheck/FaultDiagnose/CurrZeroDriftFltDiag/IvZeroDriftDiag/PowerReductionCoeffDeter/If Action Subsystem2 ==
  Action Port : ActionPort  ActionPortLabel=else
  Constant : Constant  Value=C_Flt_PowerCoeffZero_s32
  Coeff : Outport
  wires:
  Constant/1 -> Coeff/1

== system FaultCheck/FaultDiagnose/CurrZeroDriftFltDiag/IwZeroDriftDiag/Diagnose/Disable ==
  Action Port : ActionPort  ActionPortLabel=if(u1 == 0)
  Constant : Constant  Value=C_Flt_NoErr_b
  FlgOut : Outport
  wires:
  Constant/1 -> FlgOut/1

== system FaultCheck/FaultDiagnose/CurrZeroDriftFltDiag/IwZeroDriftDiag/Diagnose/Normal ==
  IwZeroDriftFltFlg : Inport
  Action Port : ActionPort  ActionPortLabel=else
  FlgOut : Outport
  wires:
  IwZeroDriftFltFlg/1 -> FlgOut/1

== system FaultCheck/FaultDiagnose/CurrZeroDriftFltDiag/IwZeroDriftDiag/Diagnose/Subsystem ==
  IwZeroDftEn : Inport
  SysSelfCheckDownFlg : Inport  Port=2
  Constant : Constant  Value=true
  Logical Operator : Logic  AllPortsSameDT=off  OutDataTypeStr=boolean
  Logical Operator1 : Logic  AllPortsSameDT=off  OutDataTypeStr=boolean
  Logical Operator2 : Logic  AllPortsSameDT=off  OutDataTypeStr=boolean
  IwZeroDriftDiagEn : Outport
  wires:
  SysSelfCheckDownFlg/1 -> Logical Operator2/2
  IwZeroDftEn/1 -> Logical Operator1/2
  Logical Operator1/1 -> Logical Operator/1
  Logical Operator2/1 -> Logical Operator/2
  Constant/1 -> Logical Operator1/1, Logical Operator2/1
  Logical Operator/1 -> IwZeroDriftDiagEn/1  "M_Flt_IwZeroDriftDiagEn_b"

== system FaultCheck/FaultDiagnose/CurrZeroDriftFltDiag/IwZeroDriftDiag/FaultLevelDeter/Normal ==
  Action Port : ActionPort  ActionPortLabel=if(u1 == 0)
  Constant : Constant  Value=C_Flt_LevelZero_u8
  IwZeroDriftFltLevel : Outport
  wires:
  Constant/1 -> IwZeroDriftFltLevel/1

== system FaultCheck/FaultDiagnose/CurrZeroDriftFltDiag/IwZeroDriftDiag/FaultLevelDeter/ZeroDriftFlt ==
  FaultLevel : Inport
  Action Port : ActionPort  ActionPortLabel=else
  IwZeroDriftFltLevel : Outport
  wires:
  FaultLevel/1 -> IwZeroDriftFltLevel/1

== system FaultCheck/FaultDiagnose/CurrZeroDriftFltDiag/IwZeroDriftDiag/PowerReductionCoeffDeter/If Action Subsystem ==
  Action Port : ActionPort  ActionPortLabel=if(u1 < 2)
  Constant : Constant  Value=C_Flt_PowerCoeffOne_s32
  Coeff : Outport
  wires:
  Constant/1 -> Coeff/1

== system FaultCheck/FaultDiagnose/CurrZeroDriftFltDiag/IwZeroDriftDiag/PowerReductionCoeffDeter/If Action Subsystem1 ==
  PowerCoeff : Inport
  Action Port : ActionPort  ActionPortLabel=elseif(u1 == 2)
  Coeff : Outport
  wires:
  PowerCoeff/1 -> Coeff/1

== system FaultCheck/FaultDiagnose/CurrZeroDriftFltDiag/IwZeroDriftDiag/PowerReductionCoeffDeter/If Action Subsystem2 ==
  Action Port : ActionPort  ActionPortLabel=else
  Constant : Constant  Value=C_Flt_PowerCoeffZero_s32
  Coeff : Outport
  wires:
  Constant/1 -> Coeff/1

== system FaultCheck/FaultDiagnose/IGBTTempDiag/IGBTULowerTempDiag/Diagnose/Disable ==
  Action Port : ActionPort  ActionPortLabel=if(u1 == 0)
  Constant : Constant  Value=C_Flt_NoErr_b
  IGBTULowerTempFltDeb : Outport
  wires:
  Constant/1 -> IGBTULowerTempFltDeb/1

== system FaultCheck/FaultDiagnose/IGBTTempDiag/IGBTULowerTempDiag/Diagnose/NormalDiag ==
  IGBTUTemp : Inport
  Parameter : Inport  Port=2
  Action Port : ActionPort  ActionPortLabel=else
  Bus Selector : BusSelector  OutputSignals=IGBTULowerTempConfirmTh,IGBTULowerTempRecoveryTh,IGBTULowerTempTrigTh,IGBTULowerTempRecTh
  DebounceRecInTwo : YS_UserDefined_Library/Fault/DebounceRecInTwo  SystemSampleTime=-1  VariantActivationTime=update diagram  Latency=0  AutoFrameSizeCalculation=off
      settings: SourceProductName=YS
  Relational Operator : RelationalOperator  Operator=>  OutDataTypeStr=boolean  RndMeth=Simplest  InputSameDT=off
  Relational Operator1 : RelationalOperator  Operator=>  OutDataTypeStr=boolean  RndMeth=Simplest  InputSameDT=off
  Signal Copy : SignalConversion  OverrideOpt=off
  IGBTULowerTempFltDeb : Outport
  wires:
  Relational Operator1/1 -> DebounceRecInTwo/4  "M_Flt_IGBTULowerTempRecFlgUnDeb_b"
  Bus Selector/4 -> Relational Operator1/2  "<IGBTULowerTempRecTh>"
  IGBTUTemp/1 -> Relational Operator1/1, Relational Operator/2
  Bus Selector/3 -> Relational Operator/1  "<IGBTULowerTempTrigTh>"
  Signal Copy/1 -> IGBTULowerTempFltDeb/1
  Relational Operator/1 -> DebounceRecInTwo/3  "M_Flt_IGBTULowerTempFltFlgUnDeb_b"
  DebounceRecInTwo/1 -> Signal Copy/1  "M_Flt_IGBTULowerTempFltFlgDeb_b"
  Bus Selector/2 -> DebounceRecInTwo/2  "<IGBTULowerTempRecoveryTh>"
  Bus Selector/1 -> DebounceRecInTwo/1  "<IGBTULowerTempConfirmTh>"
  Parameter/1 -> Bus Selector/1

== system FaultCheck/FaultDiagnose/IGBTTempDiag/IGBTULowerTempDiag/FaultLevelDeter/LowerOne ==
  FaultLevel : Inport
  Action Port : ActionPort  ActionPortLabel=else
  IGBTULowerTempFltLevel : Outport
  wires:
  FaultLevel/1 -> IGBTULowerTempFltLevel/1

== system FaultCheck/FaultDiagnose/IGBTTempDiag/IGBTULowerTempDiag/FaultLevelDeter/Normal ==
  Action Port : ActionPort  ActionPortLabel=if(u1 == 0)
  Constant : Constant  Value=C_Flt_LevelZero_u8
  IGBTULowerTempFltLevel : Outport
  wires:
  Constant/1 -> IGBTULowerTempFltLevel/1

== system FaultCheck/FaultDiagnose/IGBTTempDiag/IGBTULowerTempDiag/PowerReductionCoeffDeter/If Action Subsystem ==
  Action Port : ActionPort  ActionPortLabel=if(u1 < 2)
  Constant : Constant  Value=C_Flt_PowerCoeffOne_s32
  Coeff : Outport
  wires:
  Constant/1 -> Coeff/1

== system FaultCheck/FaultDiagnose/IGBTTempDiag/IGBTULowerTempDiag/PowerReductionCoeffDeter/If Action Subsystem1 ==
  PowerCoeff : Inport
  Action Port : ActionPort  ActionPortLabel=elseif(u1 == 2)
  Coeff : Outport
  wires:
  PowerCoeff/1 -> Coeff/1

== system FaultCheck/FaultDiagnose/IGBTTempDiag/IGBTULowerTempDiag/PowerReductionCoeffDeter/If Action Subsystem2 ==
  Action Port : ActionPort  ActionPortLabel=else
  Constant : Constant  Value=C_Flt_PowerCoeffZero_s32
  Coeff : Outport
  wires:
  Constant/1 -> Coeff/1

== system FaultCheck/FaultDiagnose/IGBTTempDiag/IGBTUOverTempDiag/Diagnose/Disable ==
  Action Port : ActionPort  ActionPortLabel=if(u1 == 0)
  Constant : Constant  Value=C_Flt_NoErr_b
  IGBTUOverTempFltDeb : Outport
  wires:
  Constant/1 -> IGBTUOverTempFltDeb/1

== system FaultCheck/FaultDiagnose/IGBTTempDiag/IGBTUOverTempDiag/Diagnose/NormalDiag ==
  IGBTUTemp : Inport
  Parameter : Inport  Port=2
  Action Port : ActionPort  ActionPortLabel=else
  Bus Selector : BusSelector  OutputSignals=IGBTUOverTempConfirmTh,IGBTUOverTempRecoveryTh,IGBTUOverTempTrigTh,IGBTUOverTempRecTh
  DebounceRecInTwo : YS_UserDefined_Library/Fault/DebounceRecInTwo  SystemSampleTime=-1  VariantActivationTime=update diagram  Latency=0  AutoFrameSizeCalculation=off
      settings: SourceProductName=YS
  Relational Operator : RelationalOperator  Operator=<  OutDataTypeStr=boolean  RndMeth=Simplest  InputSameDT=off
  Relational Operator1 : RelationalOperator  Operator=<  OutDataTypeStr=boolean  RndMeth=Simplest  InputSameDT=off
  Signal Copy : SignalConversion  OverrideOpt=off
  IGBTUOverTempFltDeb : Outport
  wires:
  Parameter/1 -> Bus Selector/1
  Bus Selector/1 -> DebounceRecInTwo/1  "<IGBTUOverTempConfirmTh>"
  Bus Selector/2 -> DebounceRecInTwo/2  "<IGBTUOverTempRecoveryTh>"
  DebounceRecInTwo/1 -> Signal Copy/1  "M_Flt_IGBTUOverTempFltFlgDeb_b"
  Relational Operator/1 -> DebounceRecInTwo/3  "M_Flt_IGBTUOverTempFltFlgUnDeb_b"
  Signal Copy/1 -> IGBTUOverTempFltDeb/1
  Bus Selector/3 -> Relational Operator/1  "<IGBTUOverTempTrigTh>"
  IGBTUTemp/1 -> Relational Operator1/1, Relational Operator/2
  Bus Selector/4 -> Relational Operator1/2  "<IGBTUOverTempRecTh>"
  Relational Operator1/1 -> DebounceRecInTwo/4  "M_Flt_IGBTUOverTempRecFlgUnDeb_b"

== system FaultCheck/FaultDiagnose/IGBTTempDiag/IGBTUOverTempDiag/FaultLevelDeter/LowerOne ==
  FaultLevel : Inport
  Action Port : ActionPort  ActionPortLabel=else
  IGBTUOverTempFltLevel : Outport
  wires:
  FaultLevel/1 -> IGBTUOverTempFltLevel/1

== system FaultCheck/FaultDiagnose/IGBTTempDiag/IGBTUOverTempDiag/FaultLevelDeter/Normal ==
  Action Port : ActionPort  ActionPortLabel=if(u1 == 0)
  Constant : Constant  Value=C_Flt_LevelZero_u8
  IGBTUOverTempFltLevel : Outport
  wires:
  Constant/1 -> IGBTUOverTempFltLevel/1

== system FaultCheck/FaultDiagnose/IGBTTempDiag/IGBTUOverTempDiag/PowerReductionCoeffDeter/If Action Subsystem ==
  Action Port : ActionPort  ActionPortLabel=if(u1 < 2)
  Constant : Constant  Value=C_Flt_PowerCoeffOne_s32
  Coeff : Outport
  wires:
  Constant/1 -> Coeff/1

== system FaultCheck/FaultDiagnose/IGBTTempDiag/IGBTUOverTempDiag/PowerReductionCoeffDeter/If Action Subsystem1 ==
  PowerCoeff : Inport
  Action Port : ActionPort  ActionPortLabel=elseif(u1 == 2)
  Coeff : Outport
  wires:
  PowerCoeff/1 -> Coeff/1

== system FaultCheck/FaultDiagnose/IGBTTempDiag/IGBTUOverTempDiag/PowerReductionCoeffDeter/If Action Subsystem2 ==
  Action Port : ActionPort  ActionPortLabel=else
  Constant : Constant  Value=C_Flt_PowerCoeffZero_s32
  Coeff : Outport
  wires:
  Constant/1 -> Coeff/1

== system FaultCheck/FaultDiagnose/IGBTTempDiag/IGBTVLowerTempDiag/Diagnose/Disable ==
  Action Port : ActionPort  ActionPortLabel=if(u1 == 0)
  Constant : Constant  Value=C_Flt_NoErr_b
  IGBTVLowerTempFltDeb : Outport
  wires:
  Constant/1 -> IGBTVLowerTempFltDeb/1
